simulink subsystem "Day6_Scenario_1"  (R2024a)
settings: Solver=VariableStepAuto  StartTime=0.0  StopTime=10.0  RelTol=1e-3
undefined symbols (not defined in the file): DiscIntNeverNeededParam, route1_waypoint, route2_waypoint, route3_waypoint
libraries: CarMaker4SL x42, simulink x1
(part 1 of 2)
settings Model: Creator=junhyung.cha  LastModifiedBy=User

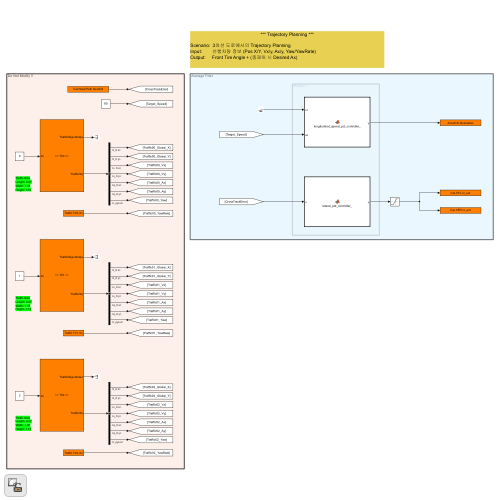
[thumbnail: Simulink's stored preview of the top-level diagram]
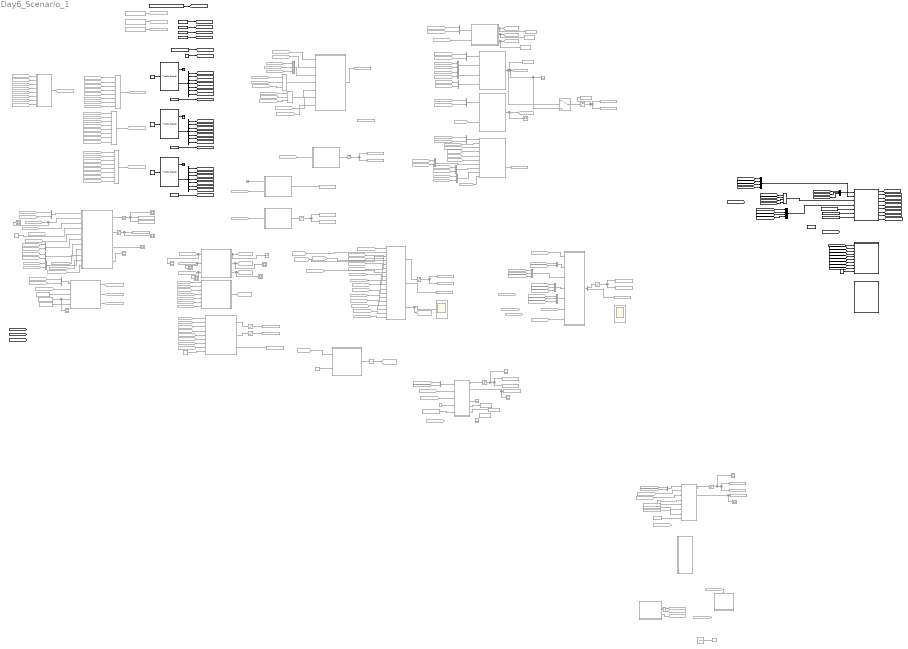
== system Day6_Scenario_1 ==
  note: Do Not Modify !!
  note: Traffic Size
      | Length: 4.47
      | Width: 1.97
      | Height: 1.12
  note: Modify !!
  note: Traffic Size
      | Length: 4.47
      | Width: 1.97
      | Height: 1.12
  note: Traffic Size
      | Length: 4.47
      | Width: 1.97
      | Height: 1.12
  note: *** Trajectory Planning ***
      |
      | Scenario: 3차선 도로에서의 Trajectory Planning
      | Input: 선행차량 정보 (Pos X/Y, Vx/y, Ax/y, Yaw/YawRate)
      | Output: Front Tire Angle + (종제어 시 Desired Ax)
  note: Modify !!
  note: Do Not Modify !!
  Bus Selector : BusSelector  OutputSignals=t_0 x,t_0 y,v_0 x,v_0 y,a_0 x,a_0 y,r_zyx z
  Bus Selector1 : BusSelector  OutputSignals=t_0 x,t_0 y,v_0 x,v_0 y,a_0 x,a_0 y,r_zyx z
  Bus Selector2 : BusSelector  OutputSignals=t_0 x,t_0 y,v_0 x,v_0 y,a_0 x,a_0 y,r_zyx z
  Chart : Stateflow chart  Commented=on  TreatAsAtomicUnit=on
  Compare To Constant : simulink/Logic and Bit Operations/Compare To Constant  Commented=on  relop=<=  const=3.0  OutDataTypeStr=boolean
  Constant : Constant  Value=80
  Constant1 : Constant  Value=0
  Constant10 : Constant  Commented=on  Value=route3_waypoint
  Constant11 : Constant  Commented=on  Value=10
  Constant12 : Constant  Commented=on  Value=route1_waypoint
  Constant13 : Constant  Commented=on  Value=10
  Constant14 : Constant  Commented=on  Value=route1_waypoint
  Constant15 : Constant  Commented=on  Value=route2_waypoint
  Constant16 : Constant  Commented=on  Value=route3_waypoint
  Constant17 : Constant  Commented=on  Value=0.001
  Constant18 : Constant
  Constant19 : Constant  Value=route1_waypoint
  Constant2 : Constant
  Constant20 : Constant  Value=route2_waypoint
  Constant21 : Constant  Value=route3_waypoint
  Constant22 : Constant  Value=0.001
  Constant3 : Constant  Value=2
  Constant4 : Constant  Commented=on  Value=20
  Constant5 : Constant  Commented=on  Value=0.001
  Constant6 : Constant  Commented=on  Value=20
  Constant7 : Constant  Value=route1_waypoint
  Constant8 : Constant  Commented=on  Value=route1_waypoint
  Constant9 : Constant  Commented=on  Value=route2_waypoint
  Demux : Demux  Commented=on  Outputs=2
  Discrete-Time Integrator : DiscreteIntegrator  Commented=on  SampleTime=-1  ICPrevOutput=DiscIntNeverNeededParam  ICPrevScaledInput=DiscIntNeverNeededParam
  From{,27,111,117,147} (5 alike) : From  Commented=on  GotoTag=Target_Speed
  From{1,14,112,118,134} (5 alike) : From  Commented=on  GotoTag=CrossTrackError
  From{10,17,45,137,149} (5 alike) : From  Commented=on  GotoTag=Traffic01_Vx
  From{2,26,34,66,100,116,146,154,159} (9 alike) : From  Commented=on  GotoTag=Ego_Vx
  From{32,63,81,101} (4 alike) : From  Commented=on  GotoTag=path_left
  From{33,64,80,102} (4 alike) : From  Commented=on  GotoTag=path_right
  From{31,62,96,103} (4 alike) : From  Commented=on  GotoTag=path_keep
  From{3,21,35,70,86,104,119,138} (8 alike) : From  Commented=on  GotoTag=Traffic00_Global_X
  From{6,22,36,71,87,105,120,139} (8 alike) : From  Commented=on  GotoTag=Traffic00_Global_Y
  From{8,24,43,88,106,121,140,144} (8 alike) : From  Commented=on  GotoTag=Traffic01_Global_X
  From{9,25,44,89,107,122,141,145} (8 alike) : From  Commented=on  GotoTag=Traffic01_Global_Y
  From{11,18,51,90,108,123,142} (7 alike) : From  Commented=on  GotoTag=Traffic02_Global_X
  From{12,19,52,91,109,124,143} (7 alike) : From  Commented=on  GotoTag=Traffic02_Global_Y
  From110 : From  Commented=on  GotoTag=best_path_idx
  From{4,15,28,67,83,92,94,97,113,125,135,152,157} (13 alike) : From  Commented=on  GotoTag=Ego_Global_X
  From{5,16,29,68,84,93,95,98,114,126,136,153,158} (13 alike) : From  Commented=on  GotoTag=Ego_Gloabl_Y
  From{30,69,82,85,99,115,127,155,160} (9 alike) : From  Commented=on  GotoTag=Ego_Yaw
  From{13,20,53,150} (4 alike) : From  Commented=on  GotoTag=Traffic02_Vx
  From130 : From  Commented=on  GotoTag=path_keep_local
  From131 : From  Commented=on  GotoTag=path_left_local
  From133 : From  Commented=on  GotoTag=path_right_local
  From{7,23,37,72,148} (5 alike) : From  Commented=on  GotoTag=Traffic00_Vx
  From151 : From  Commented=on  GotoTag=route1_waypoint
  From156 : From  Commented=on  GotoTag=route1_waypoint
  From161 : From  Commented=on  GotoTag=do_Logic
  From162 : From  Commented=on  GotoTag=do_10s
  From38 : From  Commented=on  GotoTag=Traffic00_Vy
  From39 : From  Commented=on  GotoTag=Traffic00_Ax
  From40 : From  Commented=on  GotoTag=Traffic00_Ay
  From41 : From  Commented=on  GotoTag=Traffic00_Yaw
  From42 : From  Commented=on  GotoTag=Traffic00_YawRate
  From46 : From  Commented=on  GotoTag=Traffic01_Vy
  From47 : From  Commented=on  GotoTag=Traffic01_Ax
  From48 : From  Commented=on  GotoTag=Traffic01_Ay
  From49 : From  Commented=on  GotoTag=Traffic01_Yaw
  From50 : From  Commented=on  GotoTag=Traffic01_YawRate
  From54 : From  Commented=on  GotoTag=Traffic02_Vy
  From55 : From  Commented=on  GotoTag=Traffic02_Ax
  From56 : From  Commented=on  GotoTag=Traffic02_Ay
  From57 : From  Commented=on  GotoTag=Traffic02_Yaw
  From58 : From  Commented=on  GotoTag=Traffic02_YawRate
  From59 : From  Commented=on  GotoTag=traffic2
  From60 : From  Commented=on  GotoTag=traffic0
  From61 : From  Commented=on  GotoTag=traffic1
  From65 : From  Commented=on  GotoTag=best_path_idx
  From73 : From  Commented=on  GotoTag=Traffic00_Vy
  From74 : From  Commented=on  GotoTag=Traffic00_Ax
  From75 : From  Commented=on  GotoTag=Traffic00_Ay
  From76 : From  Commented=on  GotoTag=Traffic00_Yaw
  From77 : From  Commented=on  GotoTag=Traffic00_YawRate
  From78 : From  Commented=on  GotoTag=overtake_flag
  From79 : From  Commented=on  GotoTag=best_path_idx
  Function-Call Split : FunctionCallSplit  Commented=on  IconShape=distinctive  NumOutputPorts=2  OutputPortLayout=default
  Goto : Goto  Commented=on  GotoTag=path_keep
  Goto31 : Goto  Commented=on  GotoTag=path_left
  Goto32 : Goto  Commented=on  GotoTag=path_right
  Goto33 : Goto  Commented=on  GotoTag=best_path_idx
  Goto34 : Goto  Commented=on  GotoTag=traffic0
  Goto35 : Goto  Commented=on  GotoTag=traffic1
  Goto36 : Goto  Commented=on  GotoTag=traffic2
  Goto37 : Goto  Commented=on  GotoTag=traffic0
  Goto38 : Goto  Commented=on  GotoTag=overtake_flag
  Goto39 : Goto  Commented=on  GotoTag=best_path_idx
  Goto40 : Goto  Commented=on  GotoTag=path_keep
  Goto41 : Goto  Commented=on  GotoTag=path_left
  Goto42 : Goto  Commented=on  GotoTag=path_right
  Goto43 : Goto  Commented=on  GotoTag=best_path_idx
  Goto44 : Goto  Commented=on  GotoTag=tire_angle_keep
  Goto46 : Goto  Commented=on  GotoTag=do_Logic
  Goto47 : Goto  Commented=on  GotoTag=do_Logic_
  Goto48 : Goto  Commented=on  GotoTag=do_10s
  Goto49 : Goto  Commented=on  GotoTag=path_right_local
  Goto50 : Goto  Commented=on  GotoTag=path_left_local
  Goto51 : Goto  Commented=on  GotoTag=path_keep_local
  Goto52 : Goto  Commented=on  GotoTag=route1_waypoint
  Goto53 : Goto  Commented=on  GotoTag=route2_waypoint
  Goto54 : Goto  Commented=on  GotoTag=route3_waypoint
  Ground : Ground  Commented=on
  MATLAB Function1 : MATLAB Function  Commented=on  TreatAsAtomicUnit=on
  MATLAB Function10 : MATLAB Function  Commented=on  TreatAsAtomicUnit=on
  MATLAB Function11 : MATLAB Function  Commented=on  TreatAsAtomicUnit=on
  MATLAB Function12 : MATLAB Function  Commented=on  TreatAsAtomicUnit=on
  MATLAB Function13 : MATLAB Function  Commented=on  TreatAsAtomicUnit=on
  MATLAB Function14 : MATLAB Function  Commented=on  TreatAsAtomicUnit=on
  MATLAB Function15 : MATLAB Function  Commented=on  TreatAsAtomicUnit=on
  MATLAB Function16 : MATLAB Function  Commented=on  TreatAsAtomicUnit=on
  MATLAB Function17 : MATLAB Function  Commented=on  TreatAsAtomicUnit=on
  MATLAB Function18 : MATLAB Function  Commented=on  TreatAsAtomicUnit=on
  MATLAB Function19 : MATLAB Function  Commented=on  TreatAsAtomicUnit=on
  MATLAB Function2 : MATLAB Function  Commented=on  TreatAsAtomicUnit=on
  MATLAB Function20 : MATLAB Function  Commented=on  TreatAsAtomicUnit=on
  MATLAB Function21 : MATLAB Function  TreatAsAtomicUnit=on
  MATLAB Function22 : MATLAB Function  TreatAsAtomicUnit=on
  MATLAB Function23 : MATLAB Function  TreatAsAtomicUnit=on
  MATLAB Function3 : MATLAB Function  Commented=on  TreatAsAtomicUnit=on
  MATLAB Function4 : MATLAB Function  Commented=on  TreatAsAtomicUnit=on
  MATLAB Function5 : MATLAB Function  Commented=on  TreatAsAtomicUnit=on
  MATLAB Function6 : MATLAB Function  Commented=on  TreatAsAtomicUnit=on
  MATLAB Function7 : MATLAB Function  Commented=on  TreatAsAtomicUnit=on
  MATLAB Function8 : MATLAB Function  Commented=on  TreatAsAtomicUnit=on
  MATLAB Function9 : MATLAB Function  Commented=on  TreatAsAtomicUnit=on
  Mux{,1..2,21,23..24} (6 alike) : Mux  Commented=on  Inputs=3
  Mux{3..6,10..20,22,25..26} (18 alike) : Mux  Commented=on  Inputs=2
  Mux27 : Mux  Inputs=3
  Mux28 : Mux
  Mux29 : Mux
  Mux30 : Mux
  Mux7 : Mux  Commented=on  Inputs=8
  Mux8 : Mux  Commented=on  Inputs=8
  Mux9 : Mux  Commented=on  Inputs=8
  Read CM Dict : CarMaker4SL/Read CM Dict  xname=Car.Road.Path.DevDist  xsync=off  xstime=Inherited
  Read CM Dict1 : CarMaker4SL/Read CM Dict  xname=Traffic.T00.rzv  xsync=off  xstime=Inherited
  Read CM Dict10 : CarMaker4SL/Read CM Dict  Commented=on  xname=route3_waypoint  xsync=off  xstime=Inherited
  Read CM Dict2 : CarMaker4SL/Read CM Dict  xname=Traffic.T01.rzv  xsync=off  xstime=Inherited
  Read CM Dict3 : CarMaker4SL/Read CM Dict  xname=Traffic.T02.rzv  xsync=off  xstime=Inherited
  Read CM Dict4 : CarMaker4SL/Read CM Dict  xname=Car.Fr1.tx  xsync=off  xstime=Inherited
  Read CM Dict5 : CarMaker4SL/Read CM Dict  xname=Car.Fr1.ty  xsync=off  xstime=Inherited
  Read CM Dict6 : CarMaker4SL/Read CM Dict  xname=Car.Fr1.rz  xsync=off  xstime=Inherited
  Read CM Dict7 : CarMaker4SL/Read CM Dict  xname=Car.v  xsync=off  xstime=Inherited
  Read CM Dict8 : CarMaker4SL/Read CM Dict  Commented=on  xname=route1_waypoint  xsync=off  xstime=Inherited
  Read CM Dict9 : CarMaker4SL/Read CM Dict  Commented=on  xname=route2_waypoint  xsync=off  xstime=Inherited
  Saturation{,1..5,8} (7 alike) : Saturate  Commented=on  UpperLimit=2  LowerLimit=-2
  Saturation10 : Saturate  Commented=on  UpperLimit=0.8  LowerLimit=-0.8
  Saturation6 : Saturate  Commented=on  UpperLimit=1  LowerLimit=-1
  Saturation7 : Saturate  Commented=on  UpperLimit=2  LowerLimit=-3
  Saturation9 : Saturate  Commented=on  UpperLimit=1  LowerLimit=-1
  Scope{,1..19,22..23} (22 alike) : Scope  Commented=on
  Switch : Switch  Commented=on  Threshold=1  SaturateOnIntegerOverflow=off  InputSameDT=off
  Terminator : Terminator
  Terminator1 : Terminator
  Terminator2 : Terminator
  To Workspace : ToWorkspace  Commented=on  VariableName=path_keep_out  SampleTime=-1
      settings: Save2DSignal=2-D array (concatenate along first dimension)
  To Workspace1 : ToWorkspace  Commented=on  VariableName=path_left_out  SampleTime=-1
      settings: Save2DSignal=2-D array (concatenate along first dimension)
  To Workspace2 : ToWorkspace  Commented=on  VariableName=path_right_out  SampleTime=-1
      settings: Save2DSignal=2-D array (concatenate along first dimension)
  To Workspace3 : ToWorkspace  Commented=on  VariableName=best_path_idx  SampleTime=-1
      settings: Save2DSignal=2-D array (concatenate along first dimension)
  To Workspace4 : ToWorkspace  Commented=on  VariableName=Front_Tire_Angle  SampleTime=-1
      settings: Save2DSignal=2-D array (concatenate along first dimension)
  To Workspace5 : ToWorkspace  Commented=on  VariableName=route1_xq  SaveFormat=Structure  SampleTime=-1
      settings: Save2DSignal=2-D array (concatenate along first dimension)
  To Workspace6 : ToWorkspace  Commented=on  VariableName=route1_yq  SaveFormat=Structure  SampleTime=-1
      settings: Save2DSignal=2-D array (concatenate along first dimension)
  To Workspace7 : ToWorkspace  Commented=on  VariableName=prev_idx  SampleTime=-1
      settings: Save2DSignal=2-D array (concatenate along first dimension)
  Traffic Object : CarMaker4SL/Traffic Object  xname=T00  ximode=Traffic Id  xstime=Inherited
      settings: SourceProductName=CarMaker4SL
  Traffic Object1 : CarMaker4SL/Traffic Object  xname=T01  ximode=Traffic Id  xstime=Inherited
      settings: SourceProductName=CarMaker4SL
  Traffic Object2 : CarMaker4SL/Traffic Object  xname=T02  ximode=Traffic Id  xstime=Inherited
      settings: SourceProductName=CarMaker4SL
  Triggered Subsystem : Subsystem  Commented=on  TreatAsAtomicUnit=on
  Unit Delay : UnitDelay  Commented=on  SampleTime=-1  HasFrameUpgradeWarning=on
  Write CM Dict{,4,7,10,13,16,19,22,25} (9 alike) : CarMaker4SL/Write CM Dict  Commented=on  xname=Car.CFL.rz_ext  xsync=off
  Write CM Dict{1,5,8,11,14,17,20,23,26} (9 alike) : CarMaker4SL/Write CM Dict  Commented=on  xname=Car.CFR.rz_ext  xsync=off
  Write CM Dict{2..3,6,9,12,15,18,21,24,27} (10 alike) : CarMaker4SL/Write CM Dict  Commented=on  xname=AccelCtrl.DesiredAx  xsync=off
  wires:
  Saturation/1 -> Write CM Dict1/1, Write CM Dict/1
  Constant1/1 -> Traffic Object/1
  MATLAB Function2/1(y) -> Saturation/1
  MATLAB Function1/1(y) -> Write CM Dict2/1
  From1/1 -> MATLAB Function2/1(u)
  Read CM Dict/1 -> [CrossTrackError]
  Constant/1 -> [Target_Speed]
  Bus Selector/4 -> [Traffic00_Vy]  "<v_0 y>"
  Traffic Object/1 -> Terminator/1
  Bus Selector/3 -> [Traffic00_Vx]  "<v_0 x>"
  Traffic Object/2 -> Bus Selector/1
  Bus Selector/1 -> [Traffic00_Global_X]  "<t_0 x>"
  Bus Selector/2 -> [Traffic00_Global_Y]  "<t_0 y>"
  Read CM Dict1/1 -> [Traffic00_YawRate]
  Bus Selector/5 -> [Traffic00_Ax]  "<a_0 x>"
  Bus Selector/6 -> [Traffic00_Ay]  "<a_0 y>"
  Bus Selector/7 -> [Traffic00_Yaw]  "<r_zyx z>"
  Read CM Dict2/1 -> [Traffic01_YawRate]
  Bus Selector1/1 -> [Traffic01_Global_X]  "<t_0 x>"
  Bus Selector1/5 -> [Traffic01_Ax]  "<a_0 x>"
  Bus Selector1/6 -> [Traffic01_Ay]  "<a_0 y>"
  Bus Selector1/7 -> [Traffic01_Yaw]  "<r_zyx z>"
  Traffic Object1/1 -> Terminator1/1
  Bus Selector1/4 -> [Traffic01_Vy]  "<v_0 y>"
  Constant2/1 -> Traffic Object1/1
  Traffic Object1/2 -> Bus Selector1/1
  Bus Selector1/3 -> [Traffic01_Vx]  "<v_0 x>"
  Bus Selector1/2 -> [Traffic01_Global_Y]  "<t_0 y>"
  Bus Selector2/3 -> [Traffic02_Vx]  "<v_0 x>"
  Bus Selector2/2 -> [Traffic02_Global_Y]  "<t_0 y>"
  Traffic Object2/2 -> Bus Selector2/1
  Bus Selector2/1 -> [Traffic02_Global_X]  "<t_0 x>"
  Bus Selector2/6 -> [Traffic02_Ay]  "<a_0 y>"
  Constant3/1 -> Traffic Object2/1
  Traffic Object2/1 -> Terminator2/1
  Bus Selector2/7 -> [Traffic02_Yaw]  "<r_zyx z>"
  Bus Selector2/5 -> [Traffic02_Ax]  "<a_0 x>"
  Read CM Dict3/1 -> [Traffic02_YawRate]
  Bus Selector2/4 -> [Traffic02_Vy]  "<v_0 y>"
  Read CM Dict7/1 -> [Ego_Vx]
  Read CM Dict6/1 -> [Ego_Yaw]
  Read CM Dict4/1 -> [Ego_Global_X]
  Read CM Dict5/1 -> [Ego_Gloabl_Y]
  From3/1 -> Mux/1
  From6/1 -> Mux/2
  From7/1 -> Mux/3
  From8/1 -> Mux1/1
  From9/1 -> Mux1/2
  From10/1 -> Mux1/3
  From11/1 -> Mux2/1
  From12/1 -> Mux2/2
  From13/1 -> Mux2/3
  From4/1 -> MATLAB Function1/1(ego_x)
  From5/1 -> MATLAB Function1/2(ego_y)
  Mux/1 -> MATLAB Function1/3(traffic0)
  Mux1/1 -> MATLAB Function1/4(traffic1)
  Mux2/1 -> MATLAB Function1/5(traffic2)
  From2/1 -> MATLAB Function1/6(ego_v)
  From/1 -> MATLAB Function1/7(target_speed)
  From14/1 -> MATLAB Function3/1(path_keep)
  From16/1 -> MATLAB Function3/6(ego_y)
  From15/1 -> MATLAB Function3/5(ego_x)
  From19/1 -> MATLAB Function3/15(t2_y)
  From23/1 -> MATLAB Function3/10(t0_vx)
  From20/1 -> MATLAB Function3/16(t2_vx)
  From25/1 -> MATLAB Function3/12(t1_y)
  From21/1 -> MATLAB Function3/8(t0_x)
  From22/1 -> MATLAB Function3/9(t0_y)
  From18/1 -> MATLAB Function3/14(t2_x)
  From17/1 -> MATLAB Function3/13(t1_vx)
  Saturation1/1 -> Write CM Dict4/1, Write CM Dict5/1
  MATLAB Function3/1(steer) -> Saturation1/1
  MATLAB Function3/2(accel) -> Write CM Dict6/1
  MATLAB Function4/1(path_keep) -> Goto/1, Scope/1
  MATLAB Function4/3(path_right) -> Goto32/1, Scope2/1
  From30/1 -> MATLAB Function4/3(ego_yaw), Scope5/1
  From29/1 -> MATLAB Function4/2(ego_y), Scope4/1
  From31/1 -> MATLAB Function5/1(path_keep)
  From32/1 -> MATLAB Function5/2(path_left)
  From33/1 -> MATLAB Function5/3(path_right)
  MATLAB Function6/1(traffic0) -> Goto34/1
  From35/1 -> MATLAB Function6/1(x)
  From36/1 -> MATLAB Function6/2(y)
  From37/1 -> MATLAB Function6/3(vx)
  From38/1 -> MATLAB Function6/4(vy)
  From39/1 -> MATLAB Function6/5(ax)
  From40/1 -> MATLAB Function6/6(ay)
  From41/1 -> MATLAB Function6/7(yaw)
  From42/1 -> MATLAB Function6/8(yawrate)
  From50/1 -> Mux8/8
  From49/1 -> Mux8/7
  From48/1 -> Mux8/6
  From47/1 -> Mux8/5
  From46/1 -> Mux8/4
  From45/1 -> Mux8/3
  From44/1 -> Mux8/2
  From43/1 -> Mux8/1
  Mux8/1 -> Goto35/1
  Mux9/1 -> Goto36/1
  From51/1 -> Mux9/1
  From52/1 -> Mux9/2
  From53/1 -> Mux9/3
  From54/1 -> Mux9/4
  From55/1 -> Mux9/5
  From56/1 -> Mux9/6
  From57/1 -> Mux9/7
  From58/1 -> Mux9/8
  From34/1 -> MATLAB Function5/4(ego_vx)
  From60/1 -> MATLAB Function5/5(traffic0)
  From61/1 -> MATLAB Function5/6(traffic1)
  From59/1 -> MATLAB Function5/7(traffic2)
  MATLAB Function5/1(best_path_idx) -> Goto33/1
  From64/1 -> MATLAB Function9/3(path_right)
  From63/1 -> MATLAB Function9/2(path_left)
  From62/1 -> MATLAB Function9/1(path_keep)
  From65/1 -> MATLAB Function9/4(best_path_idx)
  From67/1 -> MATLAB Function9/5(ego_x)
  From68/1 -> MATLAB Function9/6(ego_y)
  From69/1 -> MATLAB Function9/7(ego_yaw)
  From66/1 -> MATLAB Function9/8(ego_vx)
  Constant4/1 -> MATLAB Function9/9(target_speed)
  MATLAB Function9/3(DesiredAx) -> Write CM Dict9/1
  MATLAB Function9/1(steer_L) -> Saturation2/1
  MATLAB Function9/2(steer_R) -> Saturation3/1
  Saturation2/1 -> Write CM Dict7/1
  Saturation3/1 -> Write CM Dict8/1
  From77/1 -> Mux7/8
  From76/1 -> Mux7/7
  From75/1 -> Mux7/6
  From74/1 -> Mux7/5
  From73/1 -> Mux7/4
  From72/1 -> Mux7/3
  From71/1 -> Mux7/2
  From70/1 -> Mux7/1
  Mux7/1 -> Goto37/1
  MATLAB Function4/2(path_left) -> Goto31/1, Scope1/1
  From28/1 -> MATLAB Function4/1(ego_x), Scope3/1
  From27/1 -> MATLAB Function3/18(target_speed)
  From26/1 -> MATLAB Function3/17(ego_vx)
  From24/1 -> MATLAB Function3/11(t1_x)
  MATLAB Function3/3(overtake_flag) -> Goto38/1, Scope6/1
  From78/1 -> MATLAB Function7/1(overtake_flag)
  MATLAB Function7/1(best_path_idx) -> Unit Delay/1
  From79/1 -> MATLAB Function3/4(best_path_idx)
  From81/1 -> MATLAB Function3/2(path_left)
  From80/1 -> MATLAB Function3/3(path_right)
  Constant5/1 -> MATLAB Function7/2(dt)
  Unit Delay/1 -> Goto39/1
  From82/1 -> MATLAB Function3/7(ego_yaw)
  From83/1 -> Mux3/1
  From84/1 -> Mux3/2
  Mux3/1 -> MATLAB Function8/1(ego_pos)
  From85/1 -> MATLAB Function8/2(ego_yaw)
  MATLAB Function8/2(path_left_local) -> Goto41/1, To Workspace1/1
  MATLAB Function8/1(path_keep_local) -> Goto40/1, To Workspace/1
  MATLAB Function8/3(path_right_local) -> Goto42/1, To Workspace2/1
  From86/1 -> Mux4/1
  From87/1 -> Mux4/2
  From89/1 -> Mux5/2
  From88/1 -> Mux5/1
  From90/1 -> Mux6/1
  From91/1 -> Mux6/2
  Mux10/1 -> MATLAB Function10/1(ego_pos)
  From93/1 -> Mux10/2
  From92/1 -> Mux10/1
  Mux4/1 -> MATLAB Function10/2(traffic0_pos)
  Mux5/1 -> MATLAB Function10/3(traffic1_pos)
  Mux6/1 -> MATLAB Function10/4(traffic2_pos)
  From94/1 -> Mux11/1
  From95/1 -> Mux11/2
  Mux11/1 -> MATLAB Function11/1(ego_pos)
  From96/1 -> MATLAB Function11/2(path_keep)
  MATLAB Function11/1(tire_angle_keep) -> Goto44/1, Scope8/1
  Mux12/1 -> MATLAB Function12/1(ego_pos)
  From98/1 -> Mux12/2
  From97/1 -> Mux12/1
  From99/1 -> MATLAB Function12/2(ego_yaw)
  From100/1 -> MATLAB Function12/3(ego_vx)
  From103/1 -> MATLAB Function12/4(path_keep)
  From101/1 -> MATLAB Function12/5(path_left)
  From102/1 -> MATLAB Function12/6(path_right)
  Mux15/1 -> MATLAB Function12/9(traffic2_pos)
  Mux14/1 -> MATLAB Function12/8(traffic1_pos)
  Mux13/1 -> MATLAB Function12/7(traffic0_pos)
  From109/1 -> Mux15/2
  From108/1 -> Mux15/1
  From106/1 -> Mux14/1
  From107/1 -> Mux14/2
  From105/1 -> Mux13/2
  From104/1 -> Mux13/1
  From110/1 -> MATLAB Function12/10(best_path_idx)
  Saturation4/1 -> Write CM Dict11/1, Write CM Dict10/1, To Workspace4/1
  Switch/1 -> Saturation4/1
  MATLAB Function12/2(desired_ax) -> Write CM Dict12/1
  MATLAB Function10/1(best_path_idx) -> Goto43/1, Scope7/1, Switch/3, To Workspace3/1, Switch/2
  Ground/1 -> MATLAB Function13/1(u1)
  Saturation5/1 -> Write CM Dict14/1, Write CM Dict13/1
  From112/1 -> MATLAB Function14/1(u)
  MATLAB Function13/1(y) -> Write CM Dict15/1
  From111/1 -> MATLAB Function13/2(u2)
  MATLAB Function14/1(y) -> Saturation5/1
  From120/1 -> Mux17/2
  From124/1 -> Mux19/2
  From123/1 -> Mux19/1
  From119/1 -> Mux17/1
  From122/1 -> Mux18/2
  Mux17/1 -> MATLAB Function15/6(traffic0_pos)
  Mux19/1 -> MATLAB Function15/8(traffic2_pos)
  From121/1 -> Mux18/1
  From113/1 -> Mux16/1
  Mux16/1 -> MATLAB Function15/1(ego_pos)
  From114/1 -> Mux16/2
  Mux18/1 -> MATLAB Function15/7(traffic1_pos)
  From115/1 -> MATLAB Function15/2(ego_yaw), Scope13/1
  From116/1 -> MATLAB Function15/3(ego_vx)
  From118/1 -> MATLAB Function15/5(CrossTrackError)
  Saturation6/1 -> Write CM Dict16/1, Scope10/1, Write CM Dict17/1
  MATLAB Function15/2(DesiredAx) -> Saturation7/1
  MATLAB Function15/1(Front_Tire_Angle) -> Saturation6/1
  MATLAB Function15/3(cte) -> Scope9/1
  Saturation7/1 -> Write CM Dict18/1, Scope11/1
  Constant6/1 -> MATLAB Function15/4(target_speed)
  MATLAB Function15/4(best_path_idx) -> Scope12/1
  Constant7/1 -> [route1_waypoint]
  From126/1 -> Mux20/2
  Mux20/1 -> MATLAB Function17/1(ego_pos)
  From125/1 -> Mux20/1
  MATLAB Function17/1(path_keep_local) -> Goto51/1
  MATLAB Function17/2(path_left_local) -> Goto50/1
  MATLAB Function17/3(path_right_local) -> Goto49/1
  From127/1 -> MATLAB Function17/2(ego_yaw)
  Constant9/1 -> MATLAB Function17/3(route2_waypoint)
  Constant8/1 -> MATLAB Function17/4(route1_waypoint), Scope15/1
  Constant10/1 -> MATLAB Function17/5(route3_waypoint)
  Read CM Dict8/1 -> Goto52/1
  Read CM Dict9/1 -> Goto53/1
  Read CM Dict10/1 -> Goto54/1
  From130/1 -> MATLAB Function15/9(path_keep_local)
  From131/1 -> MATLAB Function15/10(path_left_local)
  From133/1 -> MATLAB Function15/11(path_right_local)
  From147/1 -> MATLAB Function16/7(Target_Speed)
  Saturation8/1 -> Write CM Dict20/1, Write CM Dict19/1
  From134/1 -> MATLAB Function16/1(CrossTrackError)
  Demux/2 -> Write CM Dict21/1
  MATLAB Function16/1(y) -> Demux/1
  Demux/1 -> Saturation8/1
  From138/1 -> Mux21/1
  From139/1 -> Mux21/2
  Mux21/1 -> MATLAB Function16/3(Traffic00)
  From141/1 -> Mux23/2
  From140/1 -> Mux23/1
  From142/1 -> Mux24/1
  From143/1 -> Mux24/2
  From148/1 -> Mux21/3
  From149/1 -> Mux23/3
  From150/1 -> Mux24/3
  Mux23/1 -> MATLAB Function16/4(Traffic01)
  Mux24/1 -> MATLAB Function16/5(Traffic02)
  From146/1 -> MATLAB Function16/6(Ego_Vx)
  Mux22/1 -> MATLAB Function16/2(Ego_XY)
  From135/1 -> Mux22/1
  From136/1 -> Mux22/2
  From153/1 -> Mux25/2
  From152/1 -> Mux25/1
  Mux25/1 -> MATLAB Function18/1(ego_pos)
  Constant12/1 -> MATLAB Function18/5(route1_waypoint)
  From155/1 -> MATLAB Function18/2(ego_yaw)
  From154/1 -> MATLAB Function18/3(ego_vx)
  Constant11/1 -> MATLAB Function18/4(target_speed)
  Saturation9/1 -> Write CM Dict23/1, Write CM Dict22/1, Scope18/1
  MATLAB Function18/1(FrontTireAngle) -> Saturation9/1
  MATLAB Function18/2(DesiredAx) -> Write CM Dict24/1, Scope19/1
  MATLAB Function18/5(route1_xq) -> To Workspace5/1
  MATLAB Function18/6(route1_yq) -> To Workspace6/1
  MATLAB Function18/4(y_local) -> Scope16/1
  ? -> To Workspace7/1
  ? -> Scope17/1
  MATLAB Function19/2(DesiredAx) -> Scope23/1, Write CM Dict27/1
  MATLAB Function19/1(FrontTireAngle) -> Saturation10/1
  Saturation10/1 -> Scope22/1, Write CM Dict25/1, Write CM Dict26/1
  Constant13/1 -> MATLAB Function19/4(target_speed)
  From159/1 -> MATLAB Function19/3(ego_vx)
  From160/1 -> MATLAB Function19/2(ego_yaw)
  Constant14/1 -> MATLAB Function19/5(route1_waypoint)
  Mux26/1 -> MATLAB Function19/1(ego_pos)
  From157/1 -> Mux26/1
  From158/1 -> Mux26/2
  Function-Call Split/2 -> Goto47/1
  Chart/1(do_Logic()) -> Function-Call Split/1
  Function-Call Split/1 -> Goto46/1
  From161/1 -> Triggered Subsystem/Trigger
  Chart/2(do_10s()) -> Goto48/1
  Discrete-Time Integrator/1 -> Compare To Constant/1
  Constant15/1 -> MATLAB Function19/6(route2_waypoint)
  Constant16/1 -> MATLAB Function19/7(route3_waypoint)
  Constant17/1 -> MATLAB Function19/8(dt)
  Constant21/1 -> MATLAB Function21/7(route3_waypoint)
  Constant20/1 -> MATLAB Function21/6(route2_waypoint)
  [Ego_Gloabl_Y] -> Mux27/2
  [Ego_Global_X] -> Mux27/1
  Mux27/1 -> MATLAB Function21/1(ego_global)
  Constant19/1 -> MATLAB Function21/5(route1_waypoint)
  [Traffic02_Vx] -> Mux30/3
  [Traffic01_Vx] -> Mux29/3
  Mux29/1 -> MATLAB Function21/3(lead2_global)
  Mux28/1 -> MATLAB Function21/2(lead1_global)
  [Traffic00_Global_X] -> Mux28/1
  [Traffic02_Global_Y] -> Mux30/2
  Mux30/1 -> MATLAB Function21/4(lead3_global)
  [Traffic01_Global_X] -> Mux29/1
  [Traffic00_Vx] -> Mux28/3
  [Traffic02_Global_X] -> Mux30/1
  [Traffic01_Global_Y] -> Mux29/2
  [Traffic00_Global_Y] -> Mux28/2
  [Ego_Yaw] -> Mux27/3
  [Traffic00_Vy] -> Mux28/4
  [Traffic01_Vy] -> Mux29/4
  [Traffic02_Vy] -> Mux30/4
  MATLAB Function21/9(route3_local) -> [route3_local]
  MATLAB Function21/6(route2_local) -> [route2_local]
  MATLAB Function21/3(route1_local) -> [route1_local]
  MATLAB Function21/8(lead_local_3) -> [lead_local_3]
  MATLAB Function21/7(ego_local_3) -> [ego_local_3]
  MATLAB Function21/5(lead_local_2) -> [lead_local_2]
  MATLAB Function21/4(ego_local_2) -> [ego_local_2]
  MATLAB Function21/2(lead_local_1) -> [lead_local_1]
  MATLAB Function21/1(ego_local_1) -> [ego_local_1]
  Constant18/1 -> MATLAB Function22/10(lane_id_in)
  [route1_local] -> MATLAB Function22/3(route1_local)
  [route3_local] -> MATLAB Function22/9(route3_local)
  [route2_local] -> MATLAB Function22/6(route2_local)
  [ego_local_1] -> MATLAB Function22/1(ego_local_1)
  [lead_local_1] -> MATLAB Function22/2(lead_local_1)
  [ego_local_2] -> MATLAB Function22/4(ego_local_2)
  [lead_local_2] -> MATLAB Function22/5(lead_local_2)
  [ego_local_3] -> MATLAB Function22/7(ego_local_3)
  [lead_local_3] -> MATLAB Function22/8(lead_local_3)

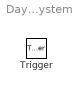
== system Day6_Scenario_1/Triggered Subsystem ==
  Trigger : TriggerPort  VariantControl=(inherit)

== matlab function Day6_Scenario_1/MATLAB Function6 ==
  settings: sampleTime=0.1
  data: x input; traffic0 output Bus: <object name>; y input; vx input; vy input; ax input; ay input; yaw input; yawrate input
function traffic0 = pack_traffic0( ...
    x, y, vx, vy, ax, ay, yaw, yawrate)

traffic0.x = x;
traffic0.y = y;
traffic0.vx = vx;
traffic0.vy = vy;
traffic0.ax = ax;
traffic0.ay = ay;
traffic0.yaw = yaw;
traffic0.yawrate = yawrate;

end

== matlab function Day6_Scenario_1/MATLAB Function7 ==
  settings: sampleTime=0.1
  data: overtake_flag input; best_path_idx output; dt input
function best_path_idx = simple_trajectory_selector(overtake_flag, dt)

persistent state timer
if isempty(state), state = 0; end
if isempty(timer), timer = 0; end

if state == 0 && overtake_flag == 1
    state = 1;
    timer = 0;
end

if state == 1
    timer = timer + dt;
    if timer > 3.0
        state = 0;
    end
end

if state == 0
    best_path_idx = 1;
else
    best_path_idx = 3;  % 추월을 오른쪽 차선 기준으로 한다면
end

end

== matlab function Day6_Scenario_1/MATLAB Function16 ==
  settings: sampleTime=0.1
  data: CrossTrackError input; Ego_XY input; Traffic00 input; Traffic01 input; Traffic02 input; Ego_Vx input; Target_Speed input; y output
function y = lateral_pid_controller_(CrossTrackError, Ego_XY, Traffic00, Traffic01, Traffic02, Ego_Vx, Target_Speed)
% 입력:
% CrossTrackError : 횡방향 오차
% Ego_XY          : [ego_x; ego_y]
% Traffic00~02    : [tx; ty; vx]
% Ego_Vx          : 자차 속도
% Target_Speed    : 목표 속도
% 출력:
% y(1): 조향각
% y(2): 종방향 가속도 명령

% ────────────── 횡방향 제어 (조향각) ──────────────
cte = CrossTrackError;

Kp_lat = 3.0;
Ki_lat = 1;
Kd_lat = 5.0;
dt     = 0.001;

persistent int_e prev_e
if isempty(int_e)
    int_e = 0;
    prev_e = 0;
end

if abs(cte) > 0.5
    int_e = int_e + cte * dt;
    d_e = (cte - prev_e) / dt;
    steer = Kp_lat * cte + Ki_lat * int_e + Kd_lat * d_e;
    steer = -steer;
    steer = max(min(steer, 0.5), -0.5);
else
    steer = 0;
end
prev_e = cte;

% ────────────── 종방향 제어 (가속도) ──────────────
ego_x = Ego_XY(1);
ego_y = Ego_XY(2);

tx0 = Traffic00(1); ty0 = Traffic00(2); vx0 = Traffic00(3);
tx1 = Traffic01(1); ty1 = Traffic01(2); vx1 = Traffic01(3);
tx2 = Traffic02(1); ty2 = Traffic02(2); vx2 = Traffic02(3);

d0 = sqrt((tx0 - ego_x)^2 + (ty0 - ego_y)^2);
d1 = sqrt((tx1 - ego_x)^2 + (ty1 - ego_y)^2);
d2 = sqrt((tx2 - ego_x)^2 + (ty2 - ego_y)^2);

[min_dist, idx] = min([d0, d1, d2]);
vx_list = [vx0, vx1, vx2];
target_v = vx_list(idx);

if min_dist < 30
    v_ref = target_v;
else
    v_ref = Target_Speed;
end

Kp_long = 2;
Kd_long = 0.1;

persistent prev_err
if isempty(prev_err)
    prev_err = 0;
end

err = v_ref - Ego_Vx;
derr = (err - prev_err) / dt;
accel = Kp_long * err + Kd_long * derr;
accel = max(min(accel, 3.0), -5.0);
prev_err = err;


% 기존 코드 ...
accel = max(min(accel, 3.0), -5.0);
prev_err = err;

% === 여기부터 속도 리미트 ===
V_MAX = 20.0; % 원하시는 값으로 조정
V_MIN = 0.0;  % 필요시 음수도 허용
v_next = Ego_Vx + accel * dt;

if v_next > V_MAX
    accel = (V_MAX - Ego_Vx) / dt;
elseif v_next < V_MIN
    accel = (V_MIN - Ego_Vx) / dt;
end


% ────────────── 출력 결합 ──────────────
y = [steer; accel];

end

== matlab function Day6_Scenario_1/MATLAB Function9 ==
  settings: sampleTime=0.1
  data: path_keep input; steer_L output size=1; path_left input; path_right input; best_path_idx input; ego_x input; ego_y input; ego_yaw input; ego_vx input; target_speed input; steer_R output size=1; DesiredAx output size=1
function [steer_L, steer_R, DesiredAx] = TrajectoryController( ...
    path_keep, path_left, path_right, ...
    best_path_idx, ...
    ego_x, ego_y, ego_yaw, ego_vx, ...
    target_speed)

% ====== 설정값 ======
LOOKAHEAD_DIST = 10.0;    % Pure Pursuit Lookahead 거리 [m]
WHEELBASE      = 2.7;     % 차량 휠베이스 [m]
Kp_ax          = 1.5;     % 종방향 제어 비례게인

% ====== 1. 최적 경로 선택 ======
if best_path_idx == 1
    path = path_keep;
elseif best_path_idx == 2
    path = path_left;
elseif best_path_idx == 3
    path = path_right;
else
    path = path_keep;  % fallback
end

% ====== 2. 조향각 계산 (Pure Pursuit) ======
dx = path(:,1) - ego_x;
dy = path(:,2) - ego_y;

cos_yaw = cos(ego_yaw);
sin_yaw = sin(ego_yaw);
x_local =  cos_yaw * dx + sin_yaw * dy;
y_local = -sin_yaw * dx + cos_yaw * dy;

% Lookahead 지점
dists = sqrt(x_local.^2 + y_local.^2);
look_idx = find(dists > LOOKAHEAD_DIST, 1);

if isempty(look_idx)
    x_look = x_local(end);
    y_look = y_local(end);
else
    x_look = x_local(look_idx);
    y_look = y_local(look_idx);
end

% 조향각 계산
alpha = atan2(y_look, x_look);
steer = atan2(2 * WHEELBASE * sin(alpha), LOOKAHEAD_DIST);

% ====== 배열 크기 명시적으로 1x1로 고정 ======
steer_L = zeros(1, 1);
steer_R = zeros(1, 1);
steer_L(1,1) = double(steer);
steer_R(1,1) = double(steer);



% ====== 3. 종방향 가속도 제어 ======
v_error = target_speed - ego_vx;
DesiredAx = double(Kp_ax * v_error);

== matlab function Day6_Scenario_1/MATLAB Function18 ==
  settings: sampleTime=0.1
  data: ego_pos input; ego_yaw input; ego_vx input; target_speed input; route1_waypoint input; FrontTireAngle output; DesiredAx output; x_local output; y_local output; route1_xq output; route1_yq output
% function [FrontTireAngle, DesiredAx, x_local, y_local] = lane_follower(ego_pos, ego_yaw, ego_vx, target_speed, route1_waypoint)
% % 입력:
% %   ego_pos         : [2x1] 또는 [1x2] 벡터, [Ego_X; Ego_Y] (Mux 입력)
% %   ego_yaw         : 차량 자세(yaw, rad)
% %   ego_vx          : 차량 속도 (m/s)
% %   target_speed    : 목표 속도 (m/s)
% %   route1_waypoint : [N x 2] 웨이포인트 (X, Y)
% % 출력:
% %   FrontTireAngle  : 조향각(rad)
% %   DesiredAx       : 가속도 명령(m/s^2)
% %   x_local, y_local: (디버깅용) 로컬 좌표상 경로점
% 
% % 1. ego_pos 분해 (Mux 입력)
% ego_x = ego_pos(1);
% ego_y = ego_pos(2);
% 
% % 2. 웨이포인트 분해 및 스플라인 보간
% x = route1_waypoint(:, 1);
% y = route1_waypoint(:, 2);
% 
% N = length(x);                % 원래 웨이포인트 개수
% t = 1:N;                      % 원본 인덱스
% tq = linspace(1, N, 10*N);    % 10배 촘촘하게 보간
% 
% route1_xq = interp1(t, x, tq, 'spline');
% route1_yq = interp1(t, y, tq, 'spline');
% 
% % 3. 모든 웨이포인트를 차량 기준 로컬 좌표로 변환
% dx_all = route1_xq - ego_x;
% dy_all = route1_yq - ego_y;
% x_local_all = dx_all * cos(-ego_yaw) - dy_all * sin(-ego_yaw);
% y_local_all = dx_all * sin(-ego_yaw) + dy_all * cos(-ego_yaw);
% 
% % 4. 차량 앞(x_local > 0) 웨이포인트만 추종
% idx_front = find(x_local_all > 0);
% if isempty(idx_front)
%     % 예외: 전부 뒤에 있으면 그냥 전체 중 최단점
%     [~, idx_min] = min(sqrt(dx_all.^2 + dy_all.^2));
% else
%     [~, idx_sub] = min(x_local_all(idx_front).^2 + y_local_all(idx_front).^2);
%     idx_min = idx_front(idx_sub);
% end
% 
% x_local = x_local_all(idx_min);
% y_local = y_local_all(idx_min);
% cte = y_local; % Cross Track Error
% 
% % --- 횡방향 PD 제어 (조향) ---
% persistent prev_e
% if isempty(prev_e)
%     prev_e = 0;
% end
% dt = 0.001;
% 
% Kp = 2.0;
% Kd = 0.1;
% 
% d_e = (cte - prev_e) / dt;
% FrontTireAngle = Kp * cte + Kd * d_e;
% prev_e = cte;
% 
% % --- 종방향 PID 제어 (속도/가속) ---
% vel_error = target_speed - ego_vx;
% persistent int_v prev_v
% if isempty(int_v)
%     int_v = 0;
%     prev_v = 0;
% end
% Kp_v = 1.2;
% Ki_v = 0.2;
% Kd_v = 0.05;
% 
% int_v = int_v + vel_error * dt;
% d_v = (vel_error - prev_v) / dt;
% DesiredAx = Kp_v * vel_error + Ki_v * int_v + Kd_v * d_v;
% prev_v = vel_error;
% 
% end



% function [FrontTireAngle, DesiredAx, x_local, y_local,route1_xq,route1_yq] = lane_follower(ego_pos, ego_yaw, ego_vx, target_speed, route1_waypoint)
% % 입력:
% %   ego_pos         : [2x1] 또는 [1x2] 벡터, [Ego_X; Ego_Y] (Mux 입력)
% %   ego_yaw         : 차량 자세(yaw, rad)
% %   ego_vx          : 차량 속도 (m/s)
% %   target_speed    : 목표 속도 (m/s)
% %   route1_waypoint : [N x 2] 웨이포인트 (X, Y)
% % 출력:
% %   FrontTireAngle  : 조향각(rad)
% %   DesiredAx       : 가속도 명령(m/s^2)
% %   x_local, y_local: (디버깅용) 로컬 좌표상 경로점
% 
% % 1. ego_pos 분해 (Mux 입력)
% ego_x = ego_pos(1);
% ego_y = ego_pos(2);
% 
% % 2. 웨이포인트 분해 및 스플라인 보간
% x = route1_waypoint(:, 1);
% y = route1_waypoint(:, 2);
% 
% N = length(x);                % 원래 웨이포인트 개수
% t = 1:N;                      % 원본 인덱스
% tq = linspace(1, N, 10*N);    % 10배 촘촘하게 보간
% 
% route1_xq = interp1(t, x, tq, 'spline');
% route1_yq = interp1(t, y, tq, 'spline');
% Nq = length(route1_xq);
% 
% % 3. (윈도우 적용) 이전 인덱스 기억
% persistent prev_idx
% if isempty(prev_idx)
%     % 첫 실행: 전체 중 가장 가까운 점
%     dist_init = sqrt((route1_xq - ego_x).^2 + (route1_yq - ego_y).^2);
%     [~, prev_idx] = min(dist_init);
% end
% 
% % 4. 윈도우 범위 지정 (이전 인덱스 기준 ±window_size)
% window_size = 20;  % 필요에 따라 조정(예: 300~1000)
% idx_min_win = max(1, prev_idx - window_size);
% idx_max_win = min(Nq, prev_idx + window_size);
% idx_win = idx_min_win:idx_max_win;
% 
% % 5. 윈도우 내 웨이포인트를 차량 기준 로컬 좌표로 변환
% dx_win = route1_xq(idx_win) - ego_x;
% dy_win = route1_yq(idx_win) - ego_y;
% x_local_win = dx_win * cos(-ego_yaw) - dy_win * sin(-ego_yaw);
% y_local_win = dx_win * sin(-ego_yaw) + dy_win * cos(-ego_yaw);
% 
% % 6. 차량 앞(x_local > 0) 웨이포인트 중에서 가장 가까운 점 추종
% idx_front = find(x_local_win > 0);
% if isempty(idx_front)
%     [~, idx_sub] = min(sqrt(dx_win.^2 + dy_win.^2));
%     idx_min = idx_win(idx_sub);
% else
%     [~, idx_sub] = min(x_local_win(idx_front).^2 + y_local_win(idx_front).^2);
%     idx_min = idx_win(idx_front(idx_sub));
% end
% 
% x_local = x_local_win(idx_min - idx_min_win + 1);
% y_local = y_local_win(idx_min - idx_min_win + 1);
% cte = y_local;
% 
% % prev_idx를 항상 최신 인덱스로 갱신
% prev_idx = idx_min;
% 
% % --- 횡방향 PD 제어 (조향) ---
% persistent prev_e
% if isempty(prev_e)
%     prev_e = 0;
% end
% dt = 0.001;
% 
% Kp = 2.0;
% Kd = 0.1;
% 
% d_e = (cte - prev_e) / dt;
% FrontTireAngle = Kp * cte + Kd * d_e;
% prev_e = cte;
% 
% % --- 종방향 PID 제어 (속도/가속) ---
% vel_error = target_speed - ego_vx;
% persistent int_v prev_v
% if isempty(int_v)
%     int_v = 0;
%     prev_v = 0;
% end
% Kp_v = 1.2;
% Ki_v = 0.2;
% Kd_v = 0.05;
% 
% int_v = int_v + vel_error * dt;
% d_v = (vel_error - prev_v) / dt;
% DesiredAx = Kp_v * vel_error + Ki_v * int_v + Kd_v * d_v;
% prev_v = vel_error;
% 
% end


% function [FrontTireAngle, DesiredAx, x_local, y_local,route1_xq,route1_yq] = lane_follower(ego_pos, ego_yaw, ego_vx, target_speed, route1_waypoint)
% % 입력:
% %   ego_pos         : [2x1] 또는 [1x2] 벡터, [Ego_X; Ego_Y] (Mux 입력)
% %   ego_yaw         : 차량 자세(yaw, rad)
% %   ego_vx          : 차량 속도 (m/s)
% %   target_speed    : 목표 속도 (m/s)
% %   route1_waypoint : [N x 2] 웨이포인트 (X, Y)
% % 출력:
% %   FrontTireAngle  : 조향각(rad)
% %   DesiredAx       : 가속도 명령(m/s^2)
% %   x_local, y_local: (디버깅용) 로컬 좌표상 경로점
% 
% % 1. ego_pos 분해 (Mux 입력)
% ego_x = ego_pos(1);
% ego_y = ego_pos(2);
% 
% % 2. 웨이포인트 분해 및 스플라인 보간
% x = route1_waypoint(:, 1);
% y = route1_waypoint(:, 2);
% 
% N = length(x);                % 원래 웨이포인트 개수
% t = 1:N;                      % 원본 인덱스
% tq = linspace(1, N, 10*N);    % 10배 촘촘하게 보간
% 
% route1_xq = interp1(t, x, tq, 'spline');
% route1_yq = interp1(t, y, tq, 'spline');
% 
% % === [중요] 보간 후 벡터로 강제 변환 (Simulink 안전)
% route1_xq = route1_xq(:);     % [Nq x 1] 열벡터
% route1_yq = route1_yq(:);     % [Nq x 1] 열벡터
% Nq = length(route1_xq);
% 
% % 3. (윈도우 적용) 이전 인덱스 기억
% persistent prev_idx
% if isempty(prev_idx)
%     dist_init = sqrt((route1_xq - ego_x).^2 + (route1_yq - ego_y).^2);
%     [~, prev_idx] = min(dist_init);
% end
% 
% % 4. 윈도우 범위 지정 (이전 인덱스 기준 ±window_size)
% window_size = 300;  % 필요에 따라 조정(예: 100~1000)
% idx_min_win = max(1, prev_idx - window_size);
% idx_max_win = min(Nq, prev_idx + window_size);
% idx_win = idx_min_win:idx_max_win;
% 
% % 5. 윈도우 내 웨이포인트를 차량 기준 로컬 좌표로 변환
% dx_win = route1_xq(idx_win) - ego_x;
% dy_win = route1_yq(idx_win) - ego_y;
% x_local_win = dx_win * cos(-ego_yaw) - dy_win * sin(-ego_yaw);
% y_local_win = dx_win * sin(-ego_yaw) + dy_win * cos(-ego_yaw);
% 
% % 6. 차량 앞(x_local > 0) 웨이포인트 중에서 가장 가까운 점 추종
% idx_front = find(x_local_win > 0);
% if isempty(idx_front)
%     [~, idx_sub] = min(sqrt(dx_win.^2 + dy_win.^2));
%     idx_min = idx_win(idx_sub);
% else
%     [~, idx_sub] = min(x_local_win(idx_front).^2 + y_local_win(idx_front).^2);
%     idx_min = idx_win(idx_front(idx_sub));
% end
% 
% x_local = x_local_win(idx_min - idx_min_win + 1);
% y_local = y_local_win(idx_min - idx_min_win + 1);
% cte = y_local;
% 
% % prev_idx를 항상 최신 인덱스로 갱신
% prev_idx = idx_min;
% 
% % --- 횡방향 PD 제어 (조향) ---
% persistent prev_e
% if isempty(prev_e)
%     prev_e = 0;
% end
% dt = 0.001;
% 
% Kp = 2.0;
% Kd = 0.1;
% 
% d_e = (cte - prev_e) / dt;
% FrontTireAngle = Kp * cte + Kd * d_e;
% prev_e = cte;
% 
% % --- 종방향 PID 제어 (속도/가속) ---
% vel_error = target_speed - ego_vx;
% persistent int_v prev_v
% if isempty(int_v)
%     int_v = 0;
%     prev_v = 0;
% end
% Kp_v = 1.2;
% Ki_v = 0.2;
% Kd_v = 0.05;
% 
% int_v = int_v + vel_error * dt;
% d_v = (vel_error - prev_v) / dt;
% DesiredAx = Kp_v * vel_error + Ki_v * int_v + Kd_v * d_v;
% prev_v = vel_error;
% 
% end


%% 1바퀴 개 잘됨

% 
% 
% function [FrontTireAngle, DesiredAx, x_local, y_local, route1_xq, route1_yq] = lane_follower(ego_pos, ego_yaw, ego_vx, target_speed, route1_waypoint)
% % 입력/출력: 동일
% 
% ego_x = ego_pos(1);
% ego_y = ego_pos(2);
% 
% % --- 1. (필수) 원본 웨이포인트가 너무 많으면 샘플링 ---
% sample_gap = 10;  % 예: 10개마다 1개 사용 (원본이 13만개면 → 1.3만개로 줄임)
% x = route1_waypoint(1:sample_gap:end,1); % [Nsamp x 1]
% y = route1_waypoint(1:sample_gap:end,2); % [Nsamp x 1]
% N = length(x);
% 
% % --- 2. 보간 배수(3~5배)로 제한, 또는 최대 1만개 ---
% interp_ratio = 3;  % 3배만 보간
% max_interp = min(10000, interp_ratio*N); % 1만개로 제한
% t = (1:N)';
% tq = linspace(1, N, max_interp)';        % [Nq x 1]
% 
% route1_xq = interp1(t, x, tq, 'spline'); % [Nq x 1] 열벡터
% route1_yq = interp1(t, y, tq, 'spline'); % [Nq x 1] 열벡터
% Nq = length(route1_xq);
% 
% % --- 3. (윈도우 적용) 이전 인덱스 기억 ---
% persistent prev_idx
% if isempty(prev_idx)
%     dist_init = sqrt((route1_xq - ego_x).^2 + (route1_yq - ego_y).^2);
%     [~, prev_idx] = min(dist_init);
% end
% 
% window_size = 300;  % 필요에 따라 조정
% idx_min_win = max(1, prev_idx - window_size);
% idx_max_win = min(Nq, prev_idx + window_size);
% idx_win = idx_min_win:idx_max_win;
% 
% dx_win = route1_xq(idx_win) - ego_x;
% dy_win = route1_yq(idx_win) - ego_y;
% x_local_win = dx_win * cos(-ego_yaw) - dy_win * sin(-ego_yaw);
% y_local_win = dx_win * sin(-ego_yaw) + dy_win * cos(-ego_yaw);
% 
% idx_front = find(x_local_win > 0);
% if isempty(idx_front)
%     [~, idx_sub] = min(sqrt(dx_win.^2 + dy_win.^2));
%     idx_min = idx_win(idx_sub);
% else
%     [~, idx_sub] = min(x_local_win(idx_front).^2 + y_local_win(idx_front).^2);
%     idx_min = idx_win(idx_front(idx_sub));
% end
% 
% x_local = x_local_win(idx_min - idx_min_win + 1);
% y_local = y_local_win(idx_min - idx_min_win + 1);
% cte = y_local;
% prev_idx = idx_min;
% 
% persistent prev_e
% if isempty(prev_e)
%     prev_e = 0;
% end
% dt = 0.001;
% Kp = 0.1;
% Kd = 0.01;
% d_e = (cte - prev_e) / dt;
% FrontTireAngle = (Kp * cte + Kd * d_e);
% prev_e = cte;
% 
% % --- 종방향 PID 제어 (속도/가속) 및 속도 리미트 ---
% vel_error = target_speed - ego_vx;
% persistent int_v prev_v
% if isempty(int_v)
%     int_v = 0;
%     prev_v = 0;
% end
% Kp_v = 1.2;
% Ki_v = 0.2;
% Kd_v = 0.05;
% int_v = int_v + vel_error * dt;
% d_v = (vel_error - prev_v) / dt;
% DesiredAx = Kp_v * vel_error + Ki_v * int_v + Kd_v * d_v;
% prev_v = vel_error;
% 
% % --- 자차 속도 리미트 (15m/s) ---
% MAX_SPEED = 15;
% if ego_vx >= MAX_SPEED && target_speed >= MAX_SPEED
%     DesiredAx = min(DesiredAx, 0); % 가속 금지, 감속만 허용
% end
% 
% end

%% 제발 연속 바퀴 돼라



function [FrontTireAngle, DesiredAx, x_local, y_local, route1_xq, route1_yq] = lane_follower(ego_pos, ego_yaw, ego_vx, target_speed, route1_waypoint)
% [무한 반복 폐곡선 주행을 위한 전체 코드]
% (1) 이상치 필터링 + (2) 폐곡선 보장 + (3) 보간 + (4) 진행방향 기반 추종

ego_x = ego_pos(1);
ego_y = ego_pos(2);

% --- 1. 샘플링 ---
sample_gap = 10;
x = route1_waypoint(1:sample_gap:end,1);
y = route1_waypoint(1:sample_gap:end,2);

% --- 2. 이상치 필터링(스파이크/점프 제거) ---
dx = diff(x); dy = diff(y);
d = sqrt(dx.^2 + dy.^2);
thresh = mean(d) + 4*std(d);    % 평균+3표준편차 (적절히 조정)
normal_idx = find([true; d < thresh]);
x_filt = x(normal_idx);
y_filt = y(normal_idx);

% --- 3. 완전한 폐곡선 보장(시작점=끝점 연결) ---
if norm([x_filt(1), y_filt(1)] - [x_filt(end), y_filt(end)]) > 1e-3
    x_filt = [x_filt; x_filt(1)];
    y_filt = [y_filt; y_filt(1)];
end

N = length(x_filt);

% --- 4. 보간 ---
interp_ratio = 3;
max_interp = min(10000, interp_ratio*N);
t = (1:N)';
tq = linspace(1, N, max_interp)';
route1_xq = interp1(t, x_filt, tq, 'spline');
route1_yq = interp1(t, y_filt, tq, 'spline');
Nq = length(route1_xq);

% --- 5. 윈도우/인덱스 관리 (폐곡선 wrap-around) ---
persistent prev_idx
if isempty(prev_idx)
    dist_init = sqrt((route1_xq - ego_x).^2 + (route1_yq - ego_y).^2);
    [~, prev_idx] = min(dist_init);
end

window_size = 300;
idx_win = mod((prev_idx-window_size):(prev_idx+window_size)-1, Nq) + 1;

dx_win = route1_xq(idx_win) - ego_x;
dy_win = route1_yq(idx_win) - ego_y;
x_local_win = dx_win * cos(-ego_yaw) - dy_win * sin(-ego_yaw);
y_local_win = dx_win * sin(-ego_yaw) + dy_win * cos(-ego_yaw);

% --- 6. 진행방향(dot product) 기반 추종점 선택 ---
Nw = length(idx_win);
tangent_vecs = zeros(Nw,2);
for i=1:Nw
    ip1 = mod(idx_win(i), Nq) + 1;
    tangent_vecs(i,1) = route1_xq(ip1) - route1_xq(idx_win(i));
    tangent_vecs(i,2) = route1_yq(ip1) - route1_yq(idx_win(i));
end
tangent_norm = sqrt(sum(tangent_vecs.^2,2));
tangent_vecs = tangent_vecs ./ max(tangent_norm, 1e-6);

ego_heading = [cos(ego_yaw), sin(ego_yaw)];
dotval = tangent_vecs * ego_heading';

valid_idx = find(x_local_win > 0 & dotval > 0.0);

if isempty(valid_idx)
    [~, idx_sub] = min(sqrt(dx_win.^2 + dy_win.^2));
    idx_min = idx_win(idx_sub);
    idx_local = idx_sub;
else
    [~, idx_sub] = min(x_local_win(valid_idx).^2 + y_local_win(valid_idx).^2);
    idx_min = idx_win(valid_idx(idx_sub));
    idx_local = valid_idx(idx_sub);
end

x_local = x_local_win(idx_local);
y_local = y_local_win(idx_local);
cte = y_local;
prev_idx = mod(idx_min - 1, Nq) + 1;

% --- 7. 횡방향 PD 제어 (조향) ---
persistent prev_e
if isempty(prev_e)
    prev_e = 0;
end
dt = 0.001;
Kp = 0.12;
Kd = 0.08;
d_e = (cte - prev_e) / dt;
FrontTireAngle = (Kp * cte + Kd * d_e); % 부호 반전 필요시 -(...)
prev_e = cte;

% --- 8. 종방향 PID 제어 (속도/가속) 및 속도 리미트 ---
vel_error = target_speed - ego_vx;
persistent int_v prev_v
if isempty(int_v)
    int_v = 0;
    prev_v = 0;
end
Kp_v = 1.2;
Ki_v = 0.2;
Kd_v = 0.05;
int_v = int_v + vel_error * dt;
d_v = (vel_error - prev_v) / dt;
DesiredAx = Kp_v * vel_error + Ki_v * int_v + Kd_v * d_v;
prev_v = vel_error;

MAX_SPEED = 15;
if ego_vx >= MAX_SPEED && target_speed >= MAX_SPEED
    DesiredAx = min(DesiredAx, 0);
end

end
